simulink library "G2ELib_V1"  (R2020b)
settings: Solver=VariableStepAuto  StartTime=0.0  StopTime=10.0  RelTol=1e-3
undefined symbols (not defined in the file or in its folder): ee_sli_rtmsupport, Filter, Filter_I_ini, Filter_V_ini, gcbh, GFM, GFM_L2, GFM_R2, Parameters_Ib, Parameters_Sb, Parameters_Un_dc, q_filter_wf, References_Q, References_Theta_Eg0, simlt, sps_rtmsupport, Vdc_loop
libraries: powerlib x48, simulink_extras x11, eeTransforms x10, pid_lib x8, spsSourcesModel x3, powerlib_meascontrol x3, spsVIMeasurementModel x3, spsFirstOrderFilterModel x3, spsSynchronousMachineModel x3, eeGeneralControl x2, eePowerMeasurement x1, sps3phSaturableTransformerModel x1
(part 1 of 5)
settings Model: Creator=keladaf  LastModifiedBy=keladaf

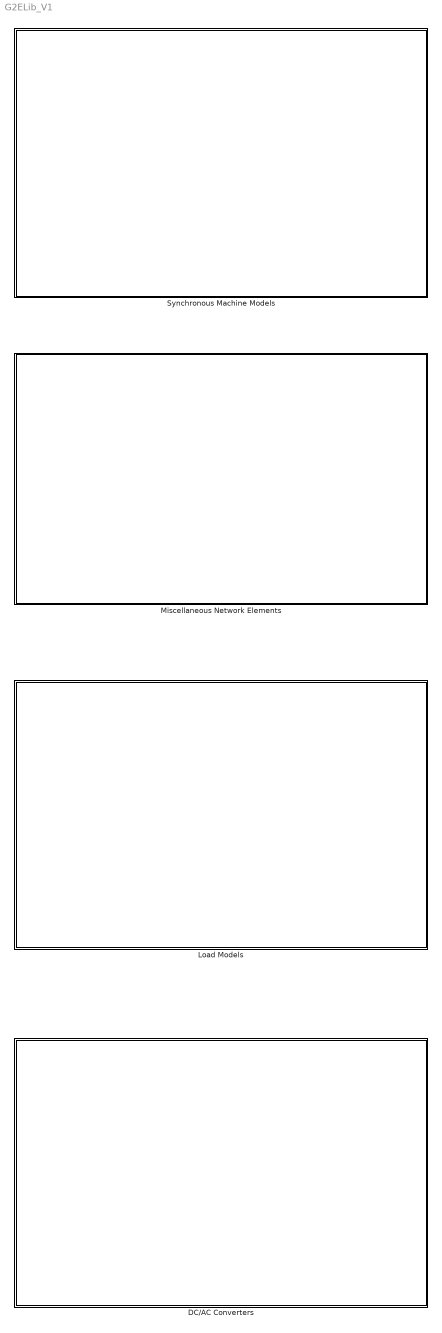
== system G2ELib_V1 ==
  DC/AC Converters : Subsystem
  Load Models : Subsystem
  Miscellaneous Network Elements : Subsystem
  Synchronous Machine Models : Subsystem

== system G2ELib_V1/DC//AC Converters ==
  Voltage Source Converters (VSC) : Subsystem

== system G2ELib_V1/Load Models ==
  note: A 3-phase Y-interconnected series RL Constant Impedance Load with an externally controlled Dynamic Load to emulate step changes in PQ of the load
  note: Don't forget to replace "i" by the actual load index {1,2,3, ...} etc
  Load_i : Subsystem
  wires:
  Load_i/1(m) -> [PQ_Loadi]

== system G2ELib_V1/Miscellaneous Network Elements ==
  note: An interconnection Bus element
  note: A 3-phase PI-section Line Model
  note: A 3-phase Y-Y Interconnection Transformer (3 single phase transformers)
      | [Per Unit Model]
  note: A Load Flow Bus To be added at each bus for load flow purposes
  note: In case Upstream Network Modelled as an Infinite Bus (Ideal three-phase voltage Source)
  Bus_i : Subsystem  DialogController=POWERSYS.PowerSysDialog  LoadFcn=|  StartFcn=sps_rtmsupport('StartFcn',gcbh);  StopFcn=sps_rtmsupport('StopFcn',gcbh);  mask(Three-Phase VI Measurement){VoltageMeasurement=phase-to-ground, SetLabelV=on, LabelV=V_Busi, Vpu=off, VpuLL=off, CurrentMeasurement=yes, SetLabelI=on, LabelI=I_Busi, Ipu=off, Pbase=100e6, Vbase=500e3, OutputType=Complex, PhasorSimulation=off, PSBequivalent=0}
      | if ~strcmp(get_param(bdroot,'BlockDiagramType'),'library')
      |     set_param([gcb,'/Model'],'LinkStatus','restore');
      | end
      | sps_rtmsupport('LoadFcn',gcbh);
      mask prompts: VoltageMeasurement "Voltage measurement"; SetLabelV "Use a label"; LabelV "Signal label  (use a From block to collect this signal)"; Vpu "Voltages in pu,  based on peak value of nominal phase-to-ground voltage"; VpuLL "Voltages in pu,  based on peak value of nominal phase-to-phase  voltage"; CurrentMeasurement "Current measurement"; SetLabelI "Use a label"; LabelI "Signal label  (use a From block to collect this signal)"; Ipu "Currents in pu"; Pbase "Base power ( VA 3 phase)"; Vbase "Nominal voltage used for pu measurement (Vrms phase-phase) :"; OutputType "Output signals in:"; PhasorSimulation "Phasor simulation (internal use)"; PSBequivalent "Equivalent circuit (internal use)"
      mask help:
      | Ideal three-phase voltage and current measurements.
      |
      | The block can output the voltages and currents in per unit values or in volts and amperes.
      mask init:
      | block = gcb;
      | Kv=1;
      | Ki=1;
      | [Kv,Ki] = powericon('ThreePhaseVIMeasurementParam',block,Vpu,VpuLL,Ipu,Vbase,Pbase,PhasorSimulation,OutputType);
      | powericon('ThreePhaseVIMeasurementCback',block);
      | power_initmask();
      settings: CopyFcn=sps_rtmsupport('CopyFcn',gcbh); powericon('ThreePhaseVIMeasurementCopy',gcb)  DeleteFcn=sps_rtmsupport('DeleteFcn',gcbh);  UndoDeleteFcn=sps_rtmsupport('UndoDeleteFcn',gcbh);  ModelCloseFcn=sps_rtmsupport('ModelCloseFcn',gcbh);  PostSaveFcn=sps_rtmsupport('PostSaveFcn',gcbh);  NameChangeFcn=sps_rtmsupport('NameChangeFcn',gcbh);  PreCopyFcn=sps_rtmsupport('PreCopyFcn',gcbh);  OpenFcn=sps_rtmsupport('OpenFcn',gcbh, [1 2 4 5 6 7 9 -12 13]);  CloseFcn=sps_rtmsupport('CloseFcn',gcbh);  PreDeleteFcn=sps_rtmsupport('PreDeleteFcn',gcbh);
      settings: PreSaveFcn=|
      | sps_rtmsupport('PreSaveFcn',gcbh);
      | if ~strcmp(get_param(bdroot(gcbh),'BlockDiagramType'),'library')
      |     set_param(gcb,'LinkStatus','restore')
      | end
      mask Help: helpview(psbhelp)
      mask TypeOptions VoltageMeasurement: no | phase-to-ground | phase-to-phase
      mask Callback VoltageMeasurement: powericon('ThreePhaseVIMeasurementCback',gcb,'Vselector');
      mask Callback SetLabelV: powericon('ThreePhaseVIMeasurementCback',gcb,'');
      mask Callback Vpu: powericon('ThreePhaseVIMeasurementCback',gcb,'Vpu');
      mask Callback VpuLL: powericon('ThreePhaseVIMeasurementCback',gcb,'VpuLL');
      mask TypeOptions CurrentMeasurement: no | yes
      mask Callback CurrentMeasurement: powericon('ThreePhaseVIMeasurementCback',gcb,'');
      mask Callback SetLabelI: powericon('ThreePhaseVIMeasurementCback',gcb,'');
      mask Callback LabelI: powericon('ThreePhaseVIMeasurementCback',gcb,'');
      mask Callback Ipu: powericon('ThreePhaseVIMeasurementCback',gcb,'');
      mask TypeOptions OutputType: Complex | Real-Imag | Magnitude-Angle | Magnitude
  Line_i : PMComponent  DialogController=POWERSYS.PowerSysDialog  LoadFcn=sps_rtmsupport('LoadFcn',gcbh);  StartFcn=sps_rtmsupport('StartFcn',gcbh);  StopFcn=sps_rtmsupport('StopFcn',gcbh);  PhysicalDomain=powersysdomain  LeftPortType=p1  RightPortType=p1  LConnTagsString=a|b|c  RConnTagsString=A|B|C  mask(Three-Phase PI Section Line){Length=1, Frequency=60, Resistances=[ 4.4965 0.3864 ], Inductances=[ 0.10103 0.0041264 ], Capacitances=[ 0.10103 7.751e-09 ]}
      mask prompts: Length "Line length (km):"; Frequency "Frequency used for rlc specification (Hz):"; Resistances "Positive- and zero-sequence resistances (Ohms/km) [ r1  r0 ]:"; Inductances "Positive- and zero-sequence inductances (H/km) [ l1  l0 ]:"; Capacitances "Positive- and zero-sequence capacitances (F/km) [ c1 c0 ]:"
      mask help:
      | This block models a three-phase transmission line with a single PI section. The model consists of one set of RL series elements connected between input and output terminals and two sets of shunt capacitances lumped at both ends of the line.
      |
      | RLC elements are computed using hyperbolic corrections yielding an exact representation in positive- and zero-sequence at specified frequency only. To obtain an extended frequency response, connect several PI section blocks in cascade or use a Distributed Parameter line.
      mask init:
      | power_initmask();
      settings: AttributesFormatString=\n  CopyFcn=sps_rtmsupport('CopyFcn',gcbh);  DeleteFcn=sps_rtmsupport('DeleteFcn',gcbh);  UndoDeleteFcn=sps_rtmsupport('UndoDeleteFcn',gcbh);  ModelCloseFcn=sps_rtmsupport('ModelCloseFcn',gcbh);  PreSaveFcn=sps_rtmsupport('PreSaveFcn',gcbh);  PostSaveFcn=sps_rtmsupport('PostSaveFcn',gcbh);  NameChangeFcn=sps_rtmsupport('NameChangeFcn',gcbh);  PreCopyFcn=sps_rtmsupport('PreCopyFcn',gcbh);  OpenFcn=sps_rtmsupport('OpenFcn',gcbh)  CloseFcn=sps_rtmsupport('CloseFcn',gcbh);  PreDeleteFcn=sps_rtmsupport('PreDeleteFcn',gcbh);
      mask Help: helpview(psbhelp);
      mask Display:
      | plot(0,0,100,100,[20,20,80,80,90,80,80,20,20,10],[50,40,40,50,50,50,61,61,50,50],[56,39],[55,55],[44,44],[44,55],[53,50,50],[44,48,55])
      | port_label('RConn', 1, 'a')
      | port_label('RConn', 2, 'b')
      | port_label('RConn', 3, 'c')
      | port_label('LConn', 1, 'A')
      | port_label('LConn', 2, 'B')
      | port_label('LConn', 3, 'C')
  Load Flow Bus : powerlib/Measurements/Load Flow Bus  LConnTagsString=a  Phases=single  Connectors=on one side  ID=BUS_1  Vbase=25e3  Vref=1  Vangle=0  VLF=1  VLFb=1  VLFc=1  angleLF=0  angleLFb=0  angleLFc=0
  Transformer_i : Subsystem  DialogController=POWERSYS.PowerSysDialog  LoadFcn=sps_rtmsupport('LoadFcn',gcbh);  StartFcn=sps_rtmsupport('StartFcn',gcbh);  StopFcn=sps_rtmsupport('StopFcn',gcbh);  mask(Three-Phase Transformer (Two Windings)){Winding1Connection=Yg, Winding2Connection=Yg, CoreType=Three single-phase transformers, SetSaturation=off, Hysteresis=off, DataFile='hysteresis', SetInitialFlux=off, Measurements=None, UNITS=pu, NominalPower=[ 100000000 60 ], Winding1=[ 230000 0 0.03125 ], Winding2=[ 18000 0 0.03125 ], Rm=500, Lm=500, L0=0.5, Saturation=[ 0,0 ; 0.0024,1.2 ; 1.0,1.52 ], InitialFluxes=[ 0.8 , -0.8 , 0.7 ], BreakLoop=off, DiscreteSolver=Trapezoidal iterative, DataType=off, TransfoNumber=1}
      mask prompts: Winding1Connection "Winding 1 connection (ABC terminals):"; Winding2Connection "Winding 2 connection (abc terminals):"; CoreType "Type:"; SetSaturation "Simulate saturation"; Hysteresis "Simulate hysteresis"; DataFile "Hysteresis Mat file (ex: 'hysteresis.mat')"; SetInitialFlux "Specify initial fluxes"; NominalPower "Nominal power and frequency  [ Pn(VA) , fn(Hz) ]"; Winding1 "Winding 1 parameters [ V1 Ph-Ph(Vrms) , R1(pu) , L1(pu) ]"; Winding2 "Winding 2 parameters [ V2 Ph-Ph(Vrms) , R2(pu) , L2(pu) ]"; Rm "Magnetization resistance  Rm (pu)"; Lm "Magnetization inductance  Lm (pu)"; L0 "Inductance L0 of zero-sequence flux path return (pu)"; Saturation "Saturation characteristic [ i1 ,  phi1 ;  i2 , phi2 ; ... ] (pu)"; InitialFluxes "Initial fluxes [ phi0A , phi0B , phi0C ] (pu):"; BreakLoop "Break Algebraic loop in discrete saturation model"; DiscreteSolver "Discrete solver model"; DataType "Use SI units (internal use)"; TransfoNumber "Device number (internal use)"
      mask help:
      | This block implements a three-phase transformer by using three single-phase transformers. Set the winding connection to 'Yn'  when you want to access the neutral point of the Wye.
      |
      | Click the Apply or the OK button after a change to the Units popup to confirm the conversion of parameters.
      mask init:
      | block = gcb;
      | [ST,Ts,WantBlockChoice] = powericon('TransformerBlocksInit','Two Windings',block,NominalPower,Winding1Connection,Winding1,Winding2Connection,Winding2,[],SetSaturation,Saturation,Hysteresis,SetInitialFlux,InitialFluxes,UNITS,DataFile,[Rm,Lm]);
      | powericon('SetInternalModels','set',block,WantBlockChoice);
      settings: CopyFcn=sps_rtmsupport('CopyFcn',gcbh); powericon('TransformerBlocksCopyFcn',gcb,3);  DeleteFcn=sps_rtmsupport('DeleteFcn',gcbh);  UndoDeleteFcn=sps_rtmsupport('UndoDeleteFcn',gcbh);  ModelCloseFcn=sps_rtmsupport('ModelCloseFcn',gcbh);  PreSaveFcn=sps_rtmsupport('PreSaveFcn',gcbh);  PostSaveFcn=sps_rtmsupport('PostSaveFcn',gcbh);  NameChangeFcn=sps_rtmsupport('NameChangeFcn',gcbh);  PreCopyFcn=sps_rtmsupport('PreCopyFcn',gcbh);  CloseFcn=sps_rtmsupport('CloseFcn',gcbh);  PreDeleteFcn=sps_rtmsupport('PreDeleteFcn',gcbh);
      settings: OpenFcn=|
      | sps_rtmsupport('OpenFcn',gcbh, [1 2 3  4 5 7  8 9 18 19 20 ]);
      | 
      | %sps_rtmsupport('OpenFcn',gcbh, [1 2 5 7 11 13 15 17]);
      mask Help: helpview(psbhelp);
      mask TypeOptions Winding1Connection: Y | Yn | Yg | Delta (D1) | Delta (D11)
      mask TypeOptions Winding2Connection: Y | Yn | Yg | Delta (D1) | Delta (D11)
      mask TypeOptions CoreType: Three single-phase transformers | Three-limb core (core-type) | Five-limb core (shell-type)
      mask Callback CoreType: powericon('ThreePhaseTransformersCback','Two Windings',gcb,'Core');
      mask Callback SetSaturation: powericon('ThreePhaseTransformersCback','Two Windings',gcb,'Saturation');
      mask Callback Hysteresis: powericon('ThreePhaseTransformersCback','Two Windings',gcb,'Hysteresis');
      mask Callback SetInitialFlux: powericon('ThreePhaseTransformersCback','Two Windings',gcb,'InitialFluxes');
      mask TypeOptions Measurements: None | Winding voltages | Winding currents | Fluxes and excitation currents ( Imag + IRm ) | Fluxes and magnetization currents ( Imag ) | All measurements (V I Fluxes)
      mask TypeOptions UNITS: SI | pu
      mask Callback UNITS: powericon('ThreePhaseTransformersCback','Two Windings',gcb,'selected units')
      mask Callback BreakLoop: powericon('ThreePhaseTransformersCback','Two Windings',gcb,'BAL');
      mask TypeOptions DiscreteSolver: Trapezoidal iterative | Trapezoidal robust | Backward Euler robust
      mask DialogControl ParameterTabVar0 Prompt: Configuration
      mask DialogControl Container6 Prompt: Core
      mask DialogControl ParameterTabVar01 Prompt: Parameters
      mask DialogControl Advanced Prompt: Advanced
      mask DialogControl Note Prompt: Specialized Power Systems can automatically handle the advanced parameters of the block. For more information, see the settings in the 'Preferences' tab of Powergui block.
      mask DialogControl Private Prompt: Internal use
      mask Display:
      | plot(-180,-220,180,220,[-100,-40],[0,0],[100,40],[0,0],[2 42 74 94 100 90 66 30 0 2 42 74 94 100 90 66 30 0 2 42 74 94 100 90 66 30 0 2 42 74 94 100 90 66 30 0]*.4-55,[-45 -45 -34 -17 3 22 38 48 50 50 55 66 83 103 122 138 148 150 150 155 166 183 203 222 238 248 250 250 255 266 283 303 322 338 348 348]*0.5-75,[2 42 74 94 100 90 66 30 0 2 42 74 94 100 90 66 30 0 2 42 74 94 100 90 66 30 0 2 42 74 94 100 90 66 30 0]*-.4+55,[-45 -45 -34 -17 3 22 38 48 50 50 55 66 83 103 122 138 148 150 150 155 166 183 203 222 238 248 250 250 255 266 283 303 322 338 348 348]*0.5-75,ST.satx,ST.saty)
      | color('gray')
      | text(ST.label1.xy(1),ST.label1.xy(2),ST.label1.name)
      | text(ST.label2.xy(1),ST.label2.xy(2),ST.label2.name)
  Upstream Network : Subsystem  DialogController=POWERSYS.PowerSysDialog  LoadFcn=sps_rtmsupport('LoadFcn',gcbh);  StartFcn=sps_rtmsupport('StartFcn',gcbh);  StopFcn=sps_rtmsupport('StopFcn',gcbh);  mask(Three-Phase Source){InternalConnection=Yg, VoltagePhases=off, Voltage=25e3, PhaseAngle=0, Voltage_phases=[25e3 25e3 25e3]/sqrt(3), PhaseAngles_phases=[0 -120 +120], Frequency=60, NonIdealSource=off, SpecifyImpedance=off, Resistance=0.8929, Inductance=16.58e-3, ShortCircuitLevel=100e6, BaseVoltage=25e3, XRratio=7, BusType=swing, Pref=10e3, Qref=0, Prefabc=[10e3, 10e3, 10e3], Qrefabc=[0, 0, 0], Qmin=-inf, Qmax=inf}
      mask prompts: InternalConnection "Configuration:"; VoltagePhases "Specify internal voltages for each phase"; Voltage "Phase-to-phase voltage (Vrms):"; PhaseAngle "Phase angle of phase A (degrees):"; Voltage_phases "Line-to-neutral voltages [Va Vb Vc] (Vrms)"; PhaseAngles_phases "Phase angle of line-to-neutral voltages [phia phib phic] (deg)"; Frequency "Frequency (Hz):"; NonIdealSource "Internal"; SpecifyImpedance "Specify short-circuit level parameters"; Resistance "Source resistance (Ohms):"; Inductance "Source inductance (H):"; ShortCircuitLevel "3-phase short-circuit level at base voltage(VA):"; BaseVoltage "Base voltage (Vrms ph-ph):"; XRratio "X/R ratio:"; BusType "Generator type:"; Pref "Active power generation P (W)"; Qref "Reactive power generation Q (var)"; Prefabc "Active power generation [Pa Pb Pc] (W)"; Qrefabc "Reactive power generation [Qa Qb Qc] (var)"; Qmin "Minimum reactive power Qmin or [Qamin,Qbmin Qcmin] (var)"; Qmax "Maximum reactive power Qmax or [Qamax,Qbmax Qcmax] (var)"
      mask help: Three-phase voltage source in series with RL branch.
      mask init:
      | block = gcb;
      | powericon('ThreePhaseSourceCback',block);
      | [s1,s2,s3,s4,g1,g2,g3,g4,g5,g6,s5] = powericon('ThreePhaseSourceIcon',SpecifyImpedance,ShortCircuitLevel,BaseVoltage,Resistance,Inductance,XRratio,InternalConnection,NonIdealSource);
      | powericon('psbloadfunction',block,'goto','Initialize');
      | [Ts, WantBlockChoice,Aa,Pa,Ab,Pb,Ac,Pc] = powericon('ThreePhaseSourceInit',block,Voltage,PhaseAngle,Voltage_phases,PhaseAngles_phases,VoltagePhases);
      | powericon('SetInternalModels','set',block,WantBlockChoice);
      settings: CopyFcn=sps_rtmsupport('CopyFcn',gcbh); powericon('psbloadfunction',gcb,'goto','UpdateGotoTag');  DeleteFcn=sps_rtmsupport('DeleteFcn',gcbh);  UndoDeleteFcn=sps_rtmsupport('UndoDeleteFcn',gcbh);  ModelCloseFcn=sps_rtmsupport('ModelCloseFcn',gcbh);  PreSaveFcn=sps_rtmsupport('PreSaveFcn',gcbh);  PostSaveFcn=sps_rtmsupport('PostSaveFcn',gcbh);  NameChangeFcn=sps_rtmsupport('NameChangeFcn',gcbh);  PreCopyFcn=sps_rtmsupport('PreCopyFcn',gcbh);  OpenFcn=sps_rtmsupport('OpenFcn',gcbh, [1,2,8,-9,15]);  CloseFcn=sps_rtmsupport('CloseFcn',gcbh);  PreDeleteFcn=sps_rtmsupport('PreDeleteFcn',gcbh);
      mask Help: helpview(psbhelp);
      mask TypeOptions InternalConnection: Y | Yn | Yg
      mask Callback InternalConnection: %powericon('ThreePhaseSourceCback',gcb);
      mask Callback VoltagePhases: powericon('ThreePhaseSourceCback',gcb);
      mask Callback NonIdealSource: powericon('ThreePhaseSourceCback',gcb);
      mask Callback SpecifyImpedance: powericon('ThreePhaseSourceCback',gcb);
      mask TypeOptions BusType: swing | PV | PQ
      mask Callback BusType: powericon('ThreePhaseSourceCback',gcb);
      mask Callback Qmax: sps_rtmsupport('parametereditingmodes',gcbh, [1,2,8,-9,15]);
      mask DialogControl Parameters Prompt: Parameters
      mask DialogControl Container7 Prompt: Source
      mask DialogControl Container6 Prompt: Impedance
      mask DialogControl LoadFlow Prompt: Load Flow
      mask Display:
      | plot(-180,-50,s5,50,s1,s2,s3,s4,[0,9,18,24,29,30,29,24,18,9,0,-9,-18,-24,-29,-30,-29,-24,-18,-9,0]*1.5-45, [30,29,24,18,9,0,-9,-18,-24,-29,-30,-29,-24,-18,-9,0,9,18,24,29,30]*0.8,[-150,-90],[0,0]);
      | plot(g1,g2,g3,g4,g5,g6);
      | plot([1 2 3 4 5 6 7 8 9 10 11 12 13 14 15 16 17 18 19 20 21].*2.5-72, [0,9,18,24,29,30,29,24,18,9,0,-9,-18,-24,-29,-30,-29,-24,-18,-9,0]./3)

== system G2ELib_V1/Synchronous Machine Models ==
  note: Rename as "SM_i" when you put in the network where "i" is the index of the SM unit {1,2,...}
  note: Proposed scope for SM units
  Bus Selector1 : BusSelector  OutputSignals=Terminal Powers (pu).Pt,References (P;V).P_ref_SM,Terminal Powers (pu).Qt,Terminal voltage dq-comp and field voltage (pu).eq,Terminal voltage dq-comp and field voltage (pu).ed,References (P;V).V_ref_SM,frequency (Hz),Load (power) angle (degrees)
  Hypot : Math  Operator=hypot  SaturateOnIntegerOverflow=on
  Mux : Mux  Inputs=2
  Mux1 : Mux  Inputs=2
  SM1_measurements : Scope  NumInputPorts=5
  Simulink - Synchronous Machine - Full Controls : Subsystem  mask{index_SM=1, SM_Sn=1e6, SM_Un=400, Parameters_fb=50, SM_wr=1, SM_Ra=0.003, SM_Ll=0.15, SM_Lad=1.66, SM_Laq=1.61, SM_L1d=0.1713, SM_R1d=0.0284, SM_L1q=0.7252, SM_R1q=0.00619, SM_L2q=0.125, SM_R2q=0.02368, SM_Rfd=0.0006, SM_Lfd=0.165, SM_H=5, SM_K_D=0, SM_Es_base=326.5986, SM_Is_base=2.0412e+03, SM_Pt=0.5, SM_Qt=0, SM_Et=1, SM_It=0.5, SM_Te_0=0.5, SM_alpha=0, SM_Phi=0.2683, SM_delta0=0.9350, SM_theta_0=-0.5597, SM_ed_0=1, SM_eq_0=0, SM_id_0=1, SM_iq_0=0, SM_efd_0=4.2550e-04, SM_ifd_0=0.7092, SM_Psi_d0=0.6545, SM_Psi_q0=-0.7580, SM_Psi_fd0=0.8149, SM_Psi_1d0=0.6978, SM_Psi_1q0=-0.6934, SM_Psi_2q0=-0.6934, SM_mp=0.5, SM_Tg=0.2, SM_Tr=20e-3, SM_Ka=300, SM_Ta=0.001, SM_Ke=1, SM_Te=0.0001, SM_Tb=0, SM_Tc=0, SM_Kf=0.001, SM_Tf=0.1, SM_Efmin=-11.5, SM_Efmax=11.5, SM_Kp=0, SM_T_LP=0.03, SM_K_PSS=2, SM_T_HP=2, SM_T1n=0.05, SM_T1d=0.02, SM_T2n=3, SM_T2d=5.4, SM_VSmax=0.15, SM_VSmin=-0.15, delta_Pref=0, T_Pref=0, delta_Vref=0, T_Vref=0}
      mask prompts: index_SM "SM index"; SM_Sn "Nominal Power (VA)"; SM_Un "Nominal Voltage (Urms)"; Parameters_fb "Nominal Frequency (Hz)"; SM_wr "Nominal Angular frequency - wr (pu)"; SM_Ra "Stator Armature Resistance (Ra - pu)"; SM_Ll "Stator Armature leakage inductance (Ll - pu)"; SM_Lad "Mutual Inductance - d-axis (Lad - pu)"; SM_Laq "Mutual Inductance - q-axis (Laq - pu)"; SM_L1d "Self inductance of amortisseur 1 circuit - d-axis (L1d - pu)"; SM_R1d "Resistance of amortisseur 1 circuit - d-axis (R1d - pu)"; SM_L1q "Self inductance of amortisseur 1 circuit - q-axis (L1q - pu)"; SM_R1q "Resistance of amortisseur 1 circuit - q-axis (R1q - pu)"; SM_L2q "Self inductance of amortisseur 2 circuit - q-axis (L2q - pu)"; SM_R2q "Resistance of amortisseur 2 circuit - q-axis (R2q - pu)"; SM_Rfd "Rotor Field Resistance - Rfd (pu)"; SM_Lfd "Rotor Field Inductance - Lfd (pu)"; SM_H "Inertia Constant - H (s)"; SM_K_D "Damping coefficient - KD (pu)"; SM_Es_base "Base Stator Voltage - Esbase (Vph - peak)"; SM_Is_base "Base Stator Current - Isbase (IL - peak)"; SM_Pt "Injected Active Power - Pt (pu)"; SM_Qt "Injected Reactive Power - Qt (pu)"; SM_Et "Terminal Voltage - Et (pu)"; SM_It "Injected Current - It (pu)"; SM_Te_0 "Initial Electrical Torque - Te0 (pu)"; SM_alpha "Voltage Phase angle - alpha (rad)"; SM_Phi "Load power factor angle - Phi (rad)"; SM_delta0 "Load angle - delta (rad)"; SM_theta_0 "initial phase shift of dq-reference frame from a-axis - theta0 (rad)"; SM_ed_0 "Initial voltage - d-axis (ed0 -pu)"; SM_eq_0 "Initial voltage - q-axis (eq0 -pu)"; SM_id_0 "Initial current - d-axis (id0 -pu)"; SM_iq_0 "Initial voltage - q-axis (iq0 -pu)"; SM_efd_0 "Initial Field Votlage - efd0 (pu)"; SM_ifd_0 "Initial Field Current - ifd0 (pu)"; SM_Psi_d0 "Initial armature circuit flux linkage - d-axis (Psid - pu)"; SM_Psi_q0 "Initial armature circuit flux linkage - q-axis (Psiq - pu)"; SM_Psi_fd0 "Initial field circuit flux linkage (Psifd - pu)"; SM_Psi_1d0 "Initial amortisseur 1 circuit flux linkage - d-axis (Psi1d - pu)"; SM_Psi_1q0 "Initial amortisseur 1 circuit flux linkage - q-axis (Psi1q - pu)"; SM_Psi_2q0 "Initial amortisseur 2 circuit flux linkage - q-axis (Psi2q - pu)"; SM_mp "Droop - mp (%)"; SM_Tg "Turbine time constant - Tg (s)"; SM_Tr "LPF time constant - Tr (s)"; SM_Ka "Regulator gain - Ka"; SM_Ta "Regulator time constant - Ta (s)"; SM_Ke "Exciter gain - Ke"; SM_Te "Exciter time constant - Te (s)"; SM_Tb "Transient gain reduction - Tb (s)"; SM_Tc "Transient gain reduction - Tc (s)"; SM_Kf "Damping filter gain (stabilizing loop)- Kf"; SM_Tf "Damping filter time constant (stabilizing loop)- Tf"; SM_Efmin "Minimum Saturation field voltage - Efmin (pu)"; SM_Efmax "Maximum Saturation field voltage - Efmax (pu)"; SM_Kp "Kp"; SM_T_LP "Sensor time constant - T_LP (s)"; SM_K_PSS "PSS Gain - K_PSS"; SM_T_HP "Wash-out time constant - T_HP (s)"; SM_T1n "Lead-lag #1 time constants - T1n"; SM_T1d "Lead-lag #1 time constants - T1d"; SM_T2n "Lead-lag #2 time constants - T2n"; SM_T2d "Lead-lag #2 time constants - T2d"; SM_VSmax "V-PSS Saturation maximum - VSmax"; SM_VSmin "V-PSS Saturation minimum - VSmin"; delta_Pref "Delta Pref (pu)"; T_Pref "Time at which the change occurs - (s)"; delta_Vref "Delta Vref (pu)"; T_Vref "Time at which the change occurs - (s)"
      settings: PortSchema="{\"entries\":[{\"content\":{\"sides\":[{\"content\":{\"connectorIds\":[\"Out1\",\"LConn1\",\"LConn2\",\"LConn3\"]},\"type\":\"ConnectorPlacement.EquallySpacedRectSide\",\"uuid\":\"d15fd8af-c839-4608-adcd-b4ba011744b3\"},{\"content\":{\"connectorIds\":[],\"side\":\"RIGHT\"},\"type\":\"ConnectorPlacement.EquallySpacedRectSide\",\"uuid\":\"fef76f33-2c1d-4a55-b0fa-e9cdd5b289ec\"},{\"content\":{\"connectorIds\":[],\"side\":\"TOP\"},\"type\":\"ConnectorPlacement.EquallySpacedRectSide\",\"uuid\":\"6886c8f2-7939-4e6f-b474-afc258dcb63b\"},{\"content\":{\"connectorIds\":[],\"side\":\"HIDDEN\"},\"type\":\"ConnectorPlacement.EquallySpacedRectSide\",\"uuid\":\"50b5083e-1b96-46a9-b16f-d88681f9c6e3\"}]},\"type\":\"ConnectorPlacement.EquallySpacedConnector\",\"uuid\":\"6c31a4b2-87e1-460a-8df1-9b61091cb655\"}],\"packageUris\":[\"http://schema.mathworks.com/mf0/Connector/R2020b\"],\"version\":\"1.0\"}"
      mask DialogControl DescTextVar Prompt: This is a full-order model of a three phase, 2-pole Synchronous Machine with two damper windings (q1 and q2) as modelled in Kundur Textbook. This also includes a simple Turbine-governor model, an IEEE Type 1 Excitation model and a Power System Stabilizer (PSS) Type 2 model.
      mask DialogControl Container10 Prompt: Parameters
      mask DialogControl ParameterGroupVar Prompt: Overview
      mask DialogControl Container5 Prompt: Nominal Values
      mask DialogControl Container6 Prompt: Electrical Parameters
      mask DialogControl Container7 Prompt: Mechanical Parameters
      mask DialogControl Container11 Prompt: Base Values
      mask DialogControl Container9 Prompt: Initializations
      mask DialogControl Container12 Prompt: Terminal Values (Load Flow)
      mask DialogControl Container14 Prompt: Angles
      mask DialogControl Container15 Prompt: dq-voltages/currents
      mask DialogControl Container16 Prompt: dq-flux linkages
      mask DialogControl Container17 Prompt: Turbine-Governor
      mask DialogControl Container18 Prompt: Exciter
      mask DialogControl Container19 Prompt: PSS
      mask DialogControl Container20 Prompt: Tests
      mask DialogControl Container21 Prompt: Reference Active Power Change
      mask DialogControl Container22 Prompt: Reference Terminal Voltage Change
      mask Display: image('$imagefile'); % Use "Edit Image" on toolstrip to change.
  wires:
  Bus Selector1/5 -> Hypot/2  "<ed>"
  Bus Selector1/2 -> Mux/2  "<P_ref_SM>"
  Bus Selector1/1 -> Mux/1  "<Pt>"
  Bus Selector1/8 -> SM1_measurements/5  "<Load (power) angle (degrees)>"
  Bus Selector1/7 -> SM1_measurements/4  "<frequency (Hz)>"
  Mux/1 -> SM1_measurements/1  "P_P_ref"
  Bus Selector1/6 -> Mux1/2  "<V_ref_SM>"
  Bus Selector1/4 -> Hypot/1  "<eq>"
  Bus Selector1/3 -> SM1_measurements/2  "<Qt>"
  Hypot/1 -> Mux1/1  "Et"
  Mux1/1 -> SM1_measurements/3  "V_V_ref"
  ? -> Bus Selector1/1
  Simulink - Synchronous Machine - Full Controls/1(m) -> [SMi_measurements]

== system G2ELib_V1/DC//AC Converters/Voltage Source Converters (VSC) ==
  Grid-Following VSC (GFL) : Subsystem
  Grid-Forming VSC (GFM) : Subsystem

== system G2ELib_V1/Load Models/Load_i ==
  Bus Creator : BusCreator  Inputs=2
  Dynamic Load : powerlib/Elements/Three-Phase Dynamic Load  NominalVoltage=[ 230000 60 ]  ActiveReactivePowers=[0 0]  PositiveSequence=[0.982229 -6.70212]  ExternalControl=on  NpNq=[1.3 2]  TimeConstants="[0  0  0  0]"  MinimumVoltage=0.7  Tfilter=1e-4  LoadFlowParameters=[4,0,0,0,0]
      settings: SourceProductBaseCode=PS
  Ground1 : powerlib/Elements/Ground  LConnTagsString=a
  Mux2 : Mux  Inputs=2
  Power Measurement (Three-Phase)1 : eePowerMeasurement/Power Measurement (Three-Phase)  LabelModeActiveChoice=Continuous  F=Parameters.fb  K=1  Seq=Positive  Ts=0
      settings: SourceProductBaseCode=PS
  Series RLC Load : powerlib/Elements/Three-Phase Series RLC Load  LConnTagsString=A|B|C  Configuration=Y (grounded)  NominalVoltage=230000  Vabc=[1e3 1e3 1e3]  Vabcp=[1e3 1e3 1e3]  NominalFrequency=60  UnbalancedPower=off  ActivePower=125000000  InductivePower=50000000  CapacitivePower=0  Pabc=[10e3 9e3 11e3]  QLabc=[100 90 110]  QCabc=[100 90 110]  Pabcp=[10e3 9e3 11e3]  QLabcp=[100 90 110]  QCabcp=[100 90 110]  Measurements=None  LoadType=constant PQ
  Step_P : Step  SampleTime=0  mask{StepV=15750000, StepT=250}
      mask prompts: StepV "Step Value (W or VAr)"; StepT "Step time (s)"
      mask DialogControl DescTextVar Prompt: A step change in active or reactive power
  Step_Q : Step  SampleTime=0  mask{StepV=1150000, StepT=500}
      mask prompts: StepV "Step Value (W or VAr)"; StepT "Step time (s)"
      mask DialogControl DescTextVar Prompt: A step change in active or reactive power
  Three-Phase Parallel RLC Branch : powerlib/Elements/Three-Phase Parallel RLC Branch  LConnTagsString=A|B|C  RConnTagsString=A|B|C  BranchType=R  Resistance=1e6  Inductance=1e-3  Capacitance=1e-6  Measurements=None
      settings: SourceProductBaseCode=PS
  Three-Phase V-I Measurement : powerlib/Measurements/Three-Phase V-I Measurement  VoltageMeasurement=phase-to-ground  SetLabelV=off  LabelV=Vabc  Vpu=off  VpuLL=off  CurrentMeasurement=yes  SetLabelI=off  LabelI=Iabc  Ipu=off  Pbase=100e6  Vbase=500e3  OutputType=Complex  PhasorSimulation=off  PSBequivalent=0
  A : PMIOPort  Side=Left
  B : PMIOPort  Port=2  Side=Left
  C : PMIOPort  Port=3  Side=Left
  m : Outport
  wires:
  Step_P/1 -> Mux2/1
  Bus Creator/1 -> m/1
  Power Measurement (Three-Phase)1/1 -> Bus Creator/1  "P_load"
  Three-Phase V-I Measurement/1 -> Power Measurement (Three-Phase)1/1
  Power Measurement (Three-Phase)1/2 -> Bus Creator/2  "Q_load"
  Step_Q/1 -> Mux2/2
  Mux2/1 -> Dynamic Load/1
  Three-Phase V-I Measurement/2 -> Power Measurement (Three-Phase)1/2
  connections:
  C/RConn1 -- Three-Phase V-I Measurement/LConn3
  A/RConn1 -- Three-Phase V-I Measurement/LConn1
  B/RConn1 -- Three-Phase V-I Measurement/LConn2
  Dynamic Load/LConn3 -- Three-Phase Parallel RLC Branch/LConn3 -- Series RLC Load/LConn3 -- Three-Phase V-I Measurement/RConn3
  Three-Phase Parallel RLC Branch/RConn1 -- Ground1/LConn1 -- Three-Phase Parallel RLC Branch/RConn2 -- Three-Phase Parallel RLC Branch/RConn3
  Series RLC Load/LConn1 -- Three-Phase Parallel RLC Branch/LConn1 -- Dynamic Load/LConn1 -- Three-Phase V-I Measurement/RConn1
  Dynamic Load/LConn2 -- Series RLC Load/LConn2 -- Three-Phase V-I Measurement/RConn2 -- Three-Phase Parallel RLC Branch/LConn2

== system G2ELib_V1/Miscellaneous Network Elements/Bus_i ==
  Kv : Gain  Gain=Ki  SaturateOnIntegerOverflow=on  OutDataTypeStr=Inherit: Same as input  ParamDataTypeStr=Inherit: Same as input
  Kv1 : Gain  Gain=Kv  SaturateOnIntegerOverflow=on  OutDataTypeStr=Inherit: Same as input  ParamDataTypeStr=Inherit: Same as input
  Mode I : spsVIMeasurementModel/Complex  SystemSampleTime=-1  VariantActivationTime=update diagram  Latency=0  AutoFrameSizeCalculation=off
      settings: SourceProductBaseCode=PS
  Mode V : spsVIMeasurementModel/Complex  SystemSampleTime=-1  VariantActivationTime=update diagram  Latency=0  AutoFrameSizeCalculation=off
      settings: SourceProductBaseCode=PS
  Model : spsVIMeasurementModel/VI  SystemSampleTime=-1  VariantActivationTime=update diagram  Latency=0  AutoFrameSizeCalculation=off
      settings: SourceProductBaseCode=PS
  A : PMIOPort  Side=Left
  B : PMIOPort  Port=2  Side=Left
  C : PMIOPort  Port=3  Side=Left
  a : PMIOPort  Port=4  Side=Right
  b : PMIOPort  Port=5  Side=Right
  c : PMIOPort  Port=6  Side=Right
  tag scope: I_Busi=global, V_Busi=global
  wires:
  Model/2 -> Kv/1
  Model/1 -> Kv1/1
  Kv/1 -> Mode I/1
  Kv1/1 -> Mode V/1
  Mode I/1 -> [I_Busi]
  Mode V/1 -> [V_Busi]
  connections:
  Model/RConn3 -- c/RConn1
  Model/RConn1 -- a/RConn1
  Model/RConn2 -- b/RConn1
  Model/LConn3 -- C/RConn1
  Model/LConn1 -- A/RConn1
  Model/LConn2 -- B/RConn1

== system G2ELib_V1/Miscellaneous Network Elements/Transformer_i ==
  From1 : Ground
  From2 : Ground
  From3 : Ground
  Goto{11..13,21..23} (6 alike) : Terminator
  I_exc1 : Ground
  I_exc2 : Ground
  I_exc3 : Ground
  Model : sps3phSaturableTransformerModel/Linear  SystemSampleTime=-1  VariantActivationTime=update diagram  Latency=0  AutoFrameSizeCalculation=off
      settings: SourceProductBaseCode=PS
  Three-PhaseTransformer : PMComponent  PhysicalDomain=powersysdomain  LeftPortType=p1  RightPortType=p1  LConnTagsString=A|B|C  RConnTagsString=a|b|c  mask(InnerPowersysBlock){}
      mask Display: disp('SPS internal use\nDo not delete')
  A : PMIOPort  Side=Left
  B : PMIOPort  Port=2  Side=Left
  C : PMIOPort  Port=3  Side=Left
  a : PMIOPort  Port=4  Side=Right
  b : PMIOPort  Port=5  Side=Right
  c : PMIOPort  Port=6  Side=Right
  wires:
  I_exc3/1 -> Model/6
  I_exc2/1 -> Model/5
  I_exc1/1 -> Model/4
  Model/1 -> Goto11/1
  From2/1 -> Model/2
  From3/1 -> Model/3
  From1/1 -> Model/1
  Model/5 -> Goto13/1
  Model/3 -> Goto12/1
  Model/2 -> Goto21/1
  Model/4 -> Goto22/1
  Model/6 -> Goto23/1
  connections:
  C/RConn1 -- Three-PhaseTransformer/LConn3
  B/RConn1 -- Three-PhaseTransformer/LConn2
  A/RConn1 -- Three-PhaseTransformer/LConn1
  c/RConn1 -- Three-PhaseTransformer/RConn3
  b/RConn1 -- Three-PhaseTransformer/RConn2
  a/RConn1 -- Three-PhaseTransformer/RConn1

== system G2ELib_V1/Miscellaneous Network Elements/Upstream Network ==
  Model : spsSourcesModel/ThreePhaseSource  SystemSampleTime=-1  VariantActivationTime=update diagram  Latency=0  AutoFrameSizeCalculation=off
      settings: SourceProductBaseCode=PS
  ThreePhaseSourceBlk : PMComponent  PhysicalDomain=powersysdomain  LeftPortType=p1  RightPortType=p1  LConnTagsString=N  RConnTagsString=A|B|C  mask(InnerPowersysBlock){}
      mask Display: disp('SPS internal use\nDo not delete')
  A : PMIOPort  Side=Right
  B : PMIOPort  Port=2  Side=Right
  C : PMIOPort  Port=3  Side=Right
  tag scope: T40_3461_3126853475583=global
  wires:
  Model/1 -> [T40_3461_3126853475583]
  connections:
  A/RConn1 -- ThreePhaseSourceBlk/RConn1
  B/RConn1 -- ThreePhaseSourceBlk/RConn2
  C/RConn1 -- ThreePhaseSourceBlk/RConn3
